simulink model "Y_FK"  (R2013a)
settings: Solver=ode45  StartTime=0.0  StopTime=inf  RelTol=1e-3
undefined symbols (not defined in the file or in its folder): ToSimulink_Y_FK_ST, ToSimulink_Y_Signals2VRML
libraries: simulink x6, vrlib x1
settings Model: Creator=Jose Angel Rangel  LastModifiedBy=root

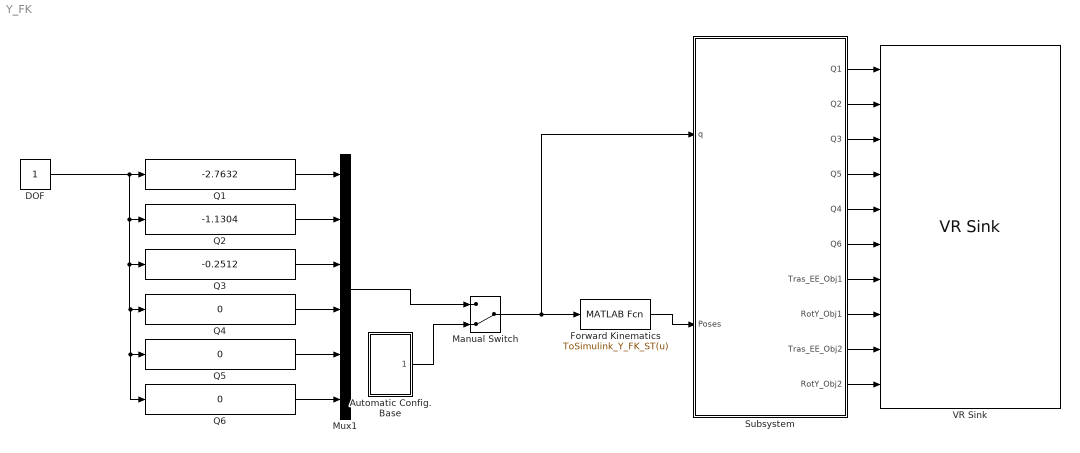
== system Y_FK ==
  Automatic Config. Base : Subsystem
  DOF : Constant
  Forward Kinematics : MATLABFcn  MATLABFcn=ToSimulink_Y_FK_ST(u)
  Manual Switch : ManualSwitch  CurrentSetting=0
  Mux1 : Mux  Inputs=6
  "Q1 " : simulink/Math Operations/Slider Gain  low=-6.28  gain=-2.7632  high=6.28
  "Q2 " : simulink/Math Operations/Slider Gain  low=-6.28  gain=-1.1304  high=6.28
  Q3 : simulink/Math Operations/Slider Gain  low=-6.28  gain=-0.2512  high=6.28
  "Q4 " : simulink/Math Operations/Slider Gain  low=-6.28  gain=0  high=6.28
  "Q5 " : simulink/Math Operations/Slider Gain  low=-6.28  gain=0  high=6.28
  Q6 : simulink/Math Operations/Slider Gain  low=-6.28  gain=0  high=6.28
  Subsystem : Subsystem
  VR Sink : vrlib/VR Sink  InstantiateOnLoad=on  SampleTime=0.1  ViewEnable=on  RemoteChange=off  RemoteView=off  FieldsWritten=Q_1.rotation.4.1.1.double#Q_2.rotation.4.1.1.double#Q_3_Der.rotation.4.1.1.double#Q_5.rotation.4.1.1.double#Q_4_Izq.rotation.4.1.1.double#Q_6.rotation.4.1.1.double#Tras_Objective1.translation.3.1.1.double#RY_Obj1.rotation.4.1.1.double#Tras_Objective2.translation.3.1.1.double#RY_Obj2.rotation.4.1.1.double  WorldFileName=Y.WRL  AutoView=on  VideoDimensions=[]  AllowVariableSize=off  FigureProperties="{'Position', 'Name', 'Viewpoint', 'CameraBound', 'CameraDirection', 'CameraPosition', 'CameraUpVector', 'ZoomFactor', 'Antialiasing', 'Headlight', 'Lighting', 'NavPanel', 'StatusBar', 'ToolBar', 'Textures', 'Transparency', 'Triad', 'Wireframe', 'NavZones', 'NavMode', 'NavSpeed', 'CaptureFileFormat', 'CaptureFileName', 'Record2DCompressMethod', 'Record2DCompressQuality', 'Record2D', 'Record2DFileName', 'Record2DFPS'; [7.6000000000000000e+01   1.1600000000000000e+02   5.7600000000000000e+02   3.8000000000000000e+02], '', '_untitled_3', 'on', [0.0000000000000000e+00   0.0000000000000000e+00  -1.0000000000000000e+00], [0.0000000000000000e+00   0.0000000000000000e+00   0.0000000000000000e+00], [0.0000000000000000e+00   1.0000000000000000e+00   0.0000000000000000e+00], [1.0000000000000000e+00], 'on', 'on', 'on', 'halfbar', 'on', 'on', 'on', 'on', 'none', 'off', 'off', 'fly', 'normal', 'tif', '%f_anim_%n.tif', 'auto', [7.5000000000000000e+01], 'off', '%f_anim_%n.avi', [1.5000000000000000e+01]}"
  wires:
  DOF/1 -> Q6/1, "Q5 "/1, "Q4 "/1, Q3/1, "Q2 "/1, "Q1 "/1
  Q6/1 -> Mux1/6
  "Q5 "/1 -> Mux1/5
  "Q4 "/1 -> Mux1/4
  Q3/1 -> Mux1/3
  "Q2 "/1 -> Mux1/2
  "Q1 "/1 -> Mux1/1
  Automatic Config. Base/1(Base config) -> Manual Switch/2
  Mux1/1 -> Manual Switch/1
  Forward Kinematics/1 -> Subsystem/2(Poses)
  Manual Switch/1 -> Subsystem/1(q), Forward Kinematics/1
  Subsystem/1(Q1) -> VR Sink/1
  Subsystem/4(Q5) -> VR Sink/4
  Subsystem/5(Q4) -> VR Sink/5
  Subsystem/6(Q6) -> VR Sink/6
  Subsystem/7(Tras_EE_Obj1) -> VR Sink/7
  Subsystem/8(RotY_Obj1) -> VR Sink/8
  Subsystem/9(Tras_EE_Obj2) -> VR Sink/9
  Subsystem/10(RotY_Obj2) -> VR Sink/10
  Subsystem/2(Q2) -> VR Sink/2
  Subsystem/3(Q3) -> VR Sink/3

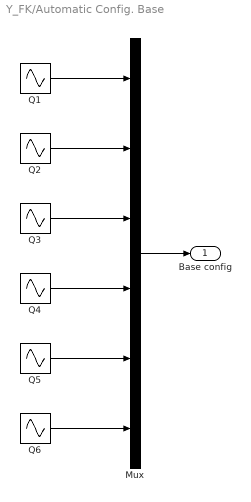
== system Y_FK/Automatic Config. Base ==
  Mux : Mux  Inputs=6
  Q1 : Sin  Amplitude=3.14  Frequency=.1  SampleTime=0
  Q2 : Sin  Amplitude=3.14  Frequency=.4  SampleTime=0
  Q3 : Sin  Amplitude=3.14  Frequency=.8  SampleTime=0
  Q4 : Sin  Amplitude=3.14  Frequency=.1  SampleTime=0
  Q5 : Sin  Amplitude=3.14  Frequency=.2  SampleTime=0
  Q6 : Sin  Amplitude=3.14  Frequency=.6  SampleTime=0
  Base config : Outport
  wires:
  Mux/1 -> Base config/1
  Q5/1 -> Mux/5
  Q6/1 -> Mux/6
  Q3/1 -> Mux/3
  Q1/1 -> Mux/1
  Q2/1 -> Mux/2
  Q4/1 -> Mux/4

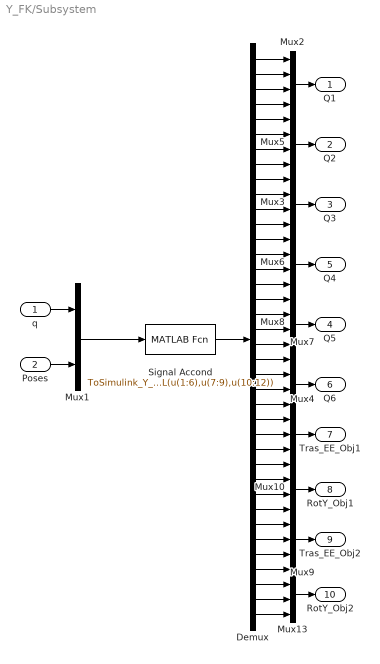
== system Y_FK/Subsystem ==
  q : Inport
  Poses : Inport  Port=2
  Demux : Demux  Outputs=38
  Mux1 : Mux  Inputs=2
  Mux{2..3,5..8,10,13} (8 alike) : Mux
  Mux4 : Mux  Inputs=3
  Mux9 : Mux  Inputs=3
  Signal Accond : MATLABFcn  MATLABFcn=ToSimulink_Y_Signals2VRML(u(1:6),u(7:9),u(10:12))
  Q1 : Outport
  Q2 : Outport  Port=2
  Q3 : Outport  Port=3
  Q5 : Outport  Port=4
  Q4 : Outport  Port=5
  Q6 : Outport  Port=6
  Tras_EE_Obj1 : Outport  Port=7
  RotY_Obj1 : Outport  Port=8
  Tras_EE_Obj2 : Outport  Port=9
  RotY_Obj2 : Outport  Port=10
  wires:
  q/1 -> Mux1/1
  Poses/1 -> Mux1/2
  Mux1/1 -> Signal Accond/1
  Signal Accond/1 -> Demux/1
  Mux2/1 -> Q1/1
  Mux5/1 -> Q2/1
  Mux3/1 -> Q3/1
  Mux6/1 -> Q4/1
  Mux8/1 -> Q5/1
  Mux7/1 -> Q6/1
  Mux4/1 -> Tras_EE_Obj1/1
  Mux10/1 -> RotY_Obj1/1
  Mux9/1 -> Tras_EE_Obj2/1
  Mux13/1 -> RotY_Obj2/1
  Demux/1 -> Mux2/1
  Demux/2 -> Mux2/2
  Demux/3 -> Mux2/3
  Demux/4 -> Mux2/4
  Demux/5 -> Mux5/1
  Demux/6 -> Mux5/2
  Demux/7 -> Mux5/3
  Demux/8 -> Mux5/4
  Demux/9 -> Mux3/1
  Demux/10 -> Mux3/2
  Demux/11 -> Mux3/3
  Demux/12 -> Mux3/4
  Demux/13 -> Mux6/1
  Demux/14 -> Mux6/2
  Demux/15 -> Mux6/3
  Demux/16 -> Mux6/4
  Demux/17 -> Mux8/1
  Demux/18 -> Mux8/2
  Demux/19 -> Mux8/3
  Demux/20 -> Mux8/4
  Demux/21 -> Mux7/1
  Demux/22 -> Mux7/2
  Demux/23 -> Mux7/3
  Demux/24 -> Mux7/4
  Demux/25 -> Mux4/1
  Demux/26 -> Mux4/2
  Demux/27 -> Mux4/3
  Demux/28 -> Mux10/1
  Demux/29 -> Mux10/2
  Demux/30 -> Mux10/3
  Demux/31 -> Mux10/4
  Demux/32 -> Mux9/1
  Demux/33 -> Mux9/2
  Demux/34 -> Mux9/3
  Demux/35 -> Mux13/1
  Demux/36 -> Mux13/2
  Demux/37 -> Mux13/3
  Demux/38 -> Mux13/4
